simulink model "N_NB_siml_robots_dyn3_general_simulink"  (R2020b)
settings: Solver=ode8  StartTime=0.0  StopTime=200  FixedStep=0.01  RelTol=1e-3
values from neighbouring files (symbols this model uses):
  A = (1/tau)*(kron(diag(r_ind_for_A1)*diag(ones(n-1,1)),[0 -tau; 0 -1])     + kron(diag((r_ind_for_A3),-1),[0 tau;0 0]))    [N_NB_siml_robots_dyn3_general.m]
  A_con = (1/h)*(-eye(n-1) + diag(ones(n-2,1),-1))    [N_NB_siml_robots_dyn3_general.m]
  B_con = zeros((n-1),1)    [N_NB_siml_robots_dyn3_general.m]
  B_u = (1/tau)*kron(eye(n-1),[0; 1])    [N_NB_siml_robots_dyn3_general.m]
  B_v = (1/tau)*[B_v_leading, B_v_init(:,idx_nonzerolines)]    [N_NB_siml_robots_dyn3_general.m]
  C = eye((n-1)*dim)    [N_NB_siml_robots_dyn3_general.m]
  C_transform_rev = [kron(eye(n-1),[1; 0])    kron(eye(n-1),[0; 1])]    [N_NB_siml_robots_dyn3_general.m]
  d = 0.1    [N_NB_siml_robots_dyn3_general.m]
  D = zeros(size(C,1),size(B_u,2))    [N_NB_siml_robots_dyn3_general.m]
  dim = 2    [N_NB_siml_robots_dyn3_general.m]
  h = 0.7    [N_NB_siml_robots_dyn3_general.m]
  kp = 0.2    [N_NB_siml_robots_dyn3_general.m]
  LR = (vehicle_length_1 + stand_still_1)*ones(n-1,1)    [N_NB_siml_robots_dyn3_general.m]
  n = 10    [N_NB_siml_robots_dyn3_general.m]
  q_initial_1 = [theta_0; s_R1_init; y_0]    [N_NB_siml_robots_dyn3_general.m]
  q_initial_2 = [theta_0; s_R2_init; y_0]    [N_NB_siml_robots_dyn3_general.m]
  q_initial_3 = [theta_0; s_R3_init; y_0]    [N_NB_siml_robots_dyn3_general.m]
  r = 0.05    [N_NB_siml_robots_dyn3_general.m]
  r_ind = zeros(1,n)    [N_NB_siml_robots_dyn3_general.m]
  robot_pos_index = [1,6,10]    [N_NB_siml_robots_dyn3_general.m]
  ur_choose_idx = find(1-r_ind)    [N_NB_siml_robots_dyn3_general.m]
  x_init = kron(d_init,[1;0]) + kron(v_init,[0;1])    [N_NB_siml_robots_dyn3_general.m]
  xc_init = zeros(n-1,1)    [N_NB_siml_robots_dyn3_general.m]
undefined symbols (not defined in the file or in its folder): C_transform
settings Model: Creator=sridhar  LastModifiedBy=sridhar

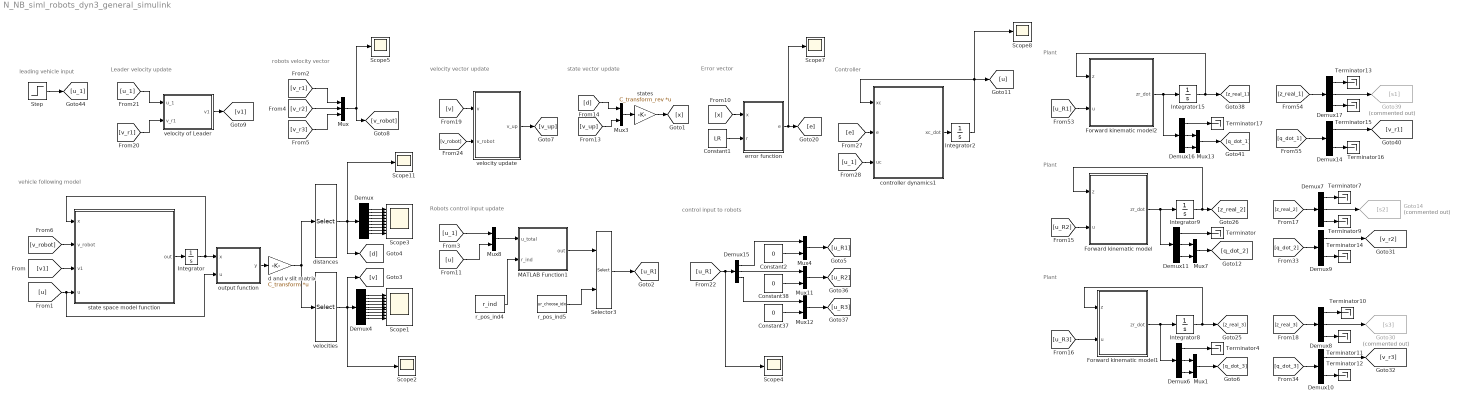
== system N_NB_siml_robots_dyn3_general_simulink ==
  note: leading vehicle input
  note: vehicle following model
  note: Leader velocity update
  note: robots velocity vector
  note: Error vector
  note: state vector update
  note: velocity vector update
  note: Robots control input update
  note: control input to robots
  note: Plant
  note: Plant
  note: Plant
  note: Controller
  Constant1 : Constant  Value=LR
  Constant2 : Constant  Value=0
  Constant37 : Constant  Value=0
  Constant38 : Constant  Value=0
  Demux : Demux  Outputs=n-1
  Demux10 : Demux  Outputs=2
  Demux{6..8,11,15..17} (7 alike) : Demux  Outputs=3
  Demux14 : Demux  Outputs=2
  Demux4 : Demux  Outputs=n-1
  Demux9 : Demux  Outputs=2
  Forward kinematic model : MATLAB Function  TreatAsAtomicUnit=on
  Forward kinematic model1 : MATLAB Function  TreatAsAtomicUnit=on
  Forward kinematic model2 : MATLAB Function  TreatAsAtomicUnit=on
  Goto14 : Goto  Commented=on  GotoTag=s2
  Goto30 : Goto  Commented=on  GotoTag=s3
  Goto39 : Goto  Commented=on  GotoTag=s1
  Integrator : Integrator  InitialCondition=x_init
  Integrator15 : Integrator  InitialCondition=q_initial_1
  Integrator2 : Integrator  InitialCondition=xc_init
  Integrator8 : Integrator  InitialCondition=q_initial_3
  Integrator9 : Integrator  InitialCondition=q_initial_2
  MATLAB Function1 : MATLAB Function  TreatAsAtomicUnit=on
  Mux : Mux  Inputs=3
  Mux{1,3..4,7..8,11..13} (8 alike) : Mux  Inputs=2
  Scope1 : Scope  NumInputPorts=9
  Scope{2,4..5,7..8,11} (6 alike) : Scope
  Scope3 : Scope  NumInputPorts=9
  Selector3 : Selector  InputPortWidth=n  IndexOptions=Index vector (port)  Indices=[1 3]  OutputSizes=1
  Step : Step  Time=100  SampleTime=0.01
  Terminator{,4,7,9..17} (12 alike) : Terminator
  controller dynamics1 : MATLAB Function  TreatAsAtomicUnit=on
  d and v slit matrix : Gain  Gain=C_transform  Multiplication=Matrix(K*u)
  distances : Selector  InputPortWidth=(n-1)*dim  IndexOptions=Index vector (dialog)  Indices=(1:n-1)  OutputSizes=1
  error function : MATLAB Function  TreatAsAtomicUnit=on
  output function : MATLAB Function  TreatAsAtomicUnit=on
  r_pos_ind4 : Constant  Value=r_ind
  r_pos_ind5 : Constant  Value=ur_choose_idx
  state space model function : MATLAB Function  TreatAsAtomicUnit=on
  states : Gain  Gain=C_transform_rev  Multiplication=Matrix(K*u)
  velocities : Selector  InputPortWidth=(n-1)*dim  IndexOptions=Index vector (dialog)  Indices=(n:dim*(n-1))  OutputSizes=1
  "velocity of Leader  " : MATLAB Function  TreatAsAtomicUnit=on
  velocity update : MATLAB Function  TreatAsAtomicUnit=on
  wires:
  Demux6/1 -> Terminator4/1
  Mux1/1 -> [q_dot_3]
  Demux6/3 -> Mux1/2
  Demux6/2 -> Mux1/1
  Integrator8/1 -> Forward kinematic model1/1(z), [z_real_3]
  Forward kinematic model1/1(zr_dot) -> Integrator8/1, Demux6/1
  [u_R3] -> Forward kinematic model1/2(u)
  [u_R2] -> Forward kinematic model/2(u)
  Forward kinematic model/1(zr_dot) -> Integrator9/1, Demux11/1
  Integrator9/1 -> [z_real_2], Forward kinematic model/1(z)
  Demux11/2 -> Mux7/1
  Demux11/3 -> Mux7/2
  Mux7/1 -> [q_dot_2]
  Demux11/1 -> Terminator/1
  Demux7/1 -> Terminator7/1
  Demux7/3 -> Terminator9/1
  Demux7/2 -> Goto14/1
  [z_real_2] -> Demux7/1
  [z_real_3] -> Demux8/1
  Demux8/2 -> Goto30/1
  Demux8/3 -> Terminator11/1
  Demux8/1 -> Terminator10/1
  Demux10/1 -> [v_r3]
  Demux10/2 -> Terminator12/1
  [q_dot_3] -> Demux10/1
  [q_dot_2] -> Demux9/1
  Demux9/2 -> Terminator14/1
  Demux9/1 -> [v_r2]
  [q_dot_1] -> Demux14/1
  Demux14/2 -> Terminator16/1
  Demux14/1 -> [v_r1]
  Demux17/1 -> Terminator13/1
  Demux17/3 -> Terminator15/1
  Demux17/2 -> Goto39/1
  [z_real_1] -> Demux17/1
  [u_R1] -> Forward kinematic model2/2(u)
  Forward kinematic model2/1(zr_dot) -> Integrator15/1, Demux16/1
  Integrator15/1 -> [z_real_1], Forward kinematic model2/1(z)
  Demux16/2 -> Mux13/1
  Demux16/3 -> Mux13/2
  Mux13/1 -> [q_dot_1]
  Demux16/1 -> Terminator17/1
  Demux15/1 -> Mux4/1
  Constant37/1 -> Mux12/2
  Constant38/1 -> Mux11/2
  [u_R] -> Scope4/1, Demux15/1
  Mux11/1 -> [u_R2]
  Constant2/1 -> Mux4/2
  Mux4/1 -> [u_R1]
  Demux15/2 -> Mux11/1
  Demux15/3 -> Mux12/1
  Mux12/1 -> [u_R3]
  velocity update/1(v_up) -> [v_up]
  [v_robot] -> velocity update/2(v_robot)
  [v] -> velocity update/1(v)
  [d] -> Mux3/1
  Mux3/1 -> states/1
  [v_up] -> Mux3/2
  states/1 -> [x]
  error function/1(e) -> Scope7/1, [e]
  [x] -> error function/1(x)
  Constant1/1 -> error function/2(r)
  [u_1] -> "velocity of Leader  "/1(u_1)
  "velocity of Leader  "/1(v1) -> [v1]
  [v_r1] -> "velocity of Leader  "/2(v_r1)
  distances/1 -> Scope11/1, Demux/1, [d]
  velocities/1 -> Scope2/1, Demux4/1, [v]
  Demux4/8 -> Scope1/8
  Demux/9 -> Scope3/9
  Demux/1 -> Scope3/1
  Demux/3 -> Scope3/3
  [v_robot] -> state space model function/2(v_robot)
  state space model function/1(out) -> Integrator/1
  output function/1(y) -> d and v slit matrix/1
  Demux/4 -> Scope3/4
  [v1] -> state space model function/3(v1)
  Demux/2 -> Scope3/2
  Demux4/2 -> Scope1/2
  Demux4/7 -> Scope1/7
  [u] -> output function/2(u), state space model function/4(u)
  Demux/7 -> Scope3/7
  Demux4/1 -> Scope1/1
  Demux/8 -> Scope3/8
  d and v slit matrix/1 -> distances/1, velocities/1
  Demux4/5 -> Scope1/5
  Demux/6 -> Scope3/6
  Demux4/3 -> Scope1/3
  Demux/5 -> Scope3/5
  Demux4/4 -> Scope1/4
  Demux4/6 -> Scope1/6
  Demux4/9 -> Scope1/9
  Integrator/1 -> output function/1(x), state space model function/1(x)
  Step/1 -> [u_1]
  [v_r2] -> Mux/2
  Mux/1 -> [v_robot], Scope5/1
  [v_r1] -> Mux/1
  [v_r3] -> Mux/3
  [e] -> controller dynamics1/2(e)
  [u_1] -> controller dynamics1/3(uc)
  controller dynamics1/1(xc_dot) -> Integrator2/1
  Integrator2/1 -> controller dynamics1/1(xc), Scope8/1, [u]
  Selector3/1 -> [u_R]
  r_pos_ind5/1 -> Selector3/2
  MATLAB Function1/1(out) -> Selector3/1
  Mux8/1 -> MATLAB Function1/1(u_total)
  [u_1] -> Mux8/1
  [u] -> Mux8/2
  r_pos_ind4/1 -> MATLAB Function1/2(r_ind)

== matlab function N_NB_siml_robots_dyn3_general_simulink/Forward kinematic model2 ==
  data: z input; u input; zr_dot output; d parameter; r parameter
function zr_dot = fcn(z,u,d,r)

%% unpacking the state vectors
theta=z(1);

%% unpacking the intput
v=u(1);
omega=u(2);

%% ODE
theta_dot=omega;
x_dot=v*cos(theta)-d*omega*sin(theta);
y_dot=v*sin(theta)+d*omega*cos(theta);
% phir_dot = (v+omega)/r;
% phil_dot = (v-omega)/r;


%% packing the output
zr_dot=[theta_dot;x_dot;y_dot];

== matlab function N_NB_siml_robots_dyn3_general_simulink/output function ==
  data: x input; u input; y output; C parameter; D parameter
function y = fcn(x,u,C, D)

y = C*x + D*u;

== matlab function N_NB_siml_robots_dyn3_general_simulink/state space model function ==
  data: x input; v_robot input; v1 input; u input; out output; A parameter; B_v parameter; B_u parameter; robot_pos_index parameter
function out = fcn(x, v_robot, v1, u, A, B_v, B_u, robot_pos_index)

if robot_pos_index(1) == 1
    v_in = v_robot;
else
    v_in = [v1; v_robot];
end
x_dot = A*x + B_u*u + B_v*v_in;
out = x_dot;

== matlab function N_NB_siml_robots_dyn3_general_simulink/MATLAB Function1 ==
  data: u_total input; out output; r_ind input
function out = fcn(u_total, r_ind)

u_dummy = diag(1-r_ind)*diag(u_total);
u_dummy_array = sum(u_dummy,2);

out = u_dummy_array;

== matlab function N_NB_siml_robots_dyn3_general_simulink/velocity update ==
  data: v input; v_robot input; v_up output; r_ind_b parameter
function v_up = fcn(v, v_robot, r_ind_b)

v_dummy = r_ind_b*v_robot;
v_up = v + v_dummy;

== matlab function N_NB_siml_robots_dyn3_general_simulink/velocity of Leader   ==
  data: u_1 input; v_r1 input; v1 output; robot_pos_index parameter
function v1 = fcn(u_1, v_r1, robot_pos_index)

if robot_pos_index(1) == 1
    v1 = v_r1;
else
    v1 = u_1;
end

== matlab function N_NB_siml_robots_dyn3_general_simulink/controller dynamics1 ==
  data: xc input; xc_dot output; e input; uc input; h parameter; A_con parameter; kp parameter; B_con parameter
function xc_dot  = fcn(xc,e,uc,h, A_con, kp, B_con)

%COMMENTS


% % control dynamics
% u1 = -kp*e(1);  % leader controller

xc_dot = A_con*xc + B_con*uc + kp/h*e;

== matlab function N_NB_siml_robots_dyn3_general_simulink/error function ==
  data: x input; e output; r input; Ce parameter
function e = fcn(x,r,Ce)

% error
e = Ce*x - r;

== matlab function N_NB_siml_robots_dyn3_general_simulink/Forward kinematic model ==
  data: z input; u input; zr_dot output; d parameter; r parameter
function zr_dot = fcn(z,u,d,r)

%% unpacking the state vectors
theta=z(1);

%% unpacking the intput
v=u(1);
omega=u(2);

%% ODE
theta_dot=omega;
x_dot=v*cos(theta)-d*omega*sin(theta);
y_dot=v*sin(theta)+d*omega*cos(theta);
% phir_dot = (v+omega)/r;
% phil_dot = (v-omega)/r;


%% packing the output
zr_dot=[theta_dot;x_dot;y_dot];

== matlab function N_NB_siml_robots_dyn3_general_simulink/Forward kinematic model1 ==
  data: z input; u input; zr_dot output; d parameter; r parameter
function zr_dot = fcn(z,u,d,r)

%% unpacking the state vectors
theta=z(1);

%% unpacking the intput
v=u(1);
omega=u(2);

%% ODE
theta_dot=omega;
x_dot=v*cos(theta)-d*omega*sin(theta);
y_dot=v*sin(theta)+d*omega*cos(theta);
% phir_dot = (v+omega)/r;
% phil_dot = (v-omega)/r;


%% packing the output
zr_dot=[theta_dot;x_dot;y_dot];
